simulink model "D53_LKAS"  (R2018b)
settings: Solver=ode3  StartTime=0.0  StopTime=10.0  FixedStep=0.01  RelTol=1e-3  EnableMultiTasking=on
model workspace (MAT data in the model file):
  MCOS : class17 (value not decoded)
  MCOS : class17 (value not decoded)
  MCOS : class17 (value not decoded)
  MCOS : class17 (value not decoded)
  MCOS : class17 (value not decoded)
  MCOS : class17 (value not decoded)
  MCOS : class17 (value not decoded)
  MCOS : class17 (value not decoded)
  MCOS : class17 (value not decoded)
  MCOS : class17 (value not decoded)
  MCOS : class17 (value not decoded)
  MCOS : class17 (value not decoded)
  MCOS : class17 (value not decoded)
  MCOS : class17 (value not decoded)
  MCOS : class17 (value not decoded)
  MCOS : class17 (value not decoded)
  MCOS : class17 (value not decoded)
  MCOS : class17 (value not decoded)
  MCOS : class17 (value not decoded)
  MCOS : class17 (value not decoded)
  MCOS : class17 (value not decoded)
  MCOS : class17 (value not decoded)
  MCOS : class17 (value not decoded)
  MCOS : class17 (value not decoded)
  MCOS : class17 (value not decoded)
  MCOS : class17 (value not decoded)
  MCOS : class17 (value not decoded)
  MCOS : class17 (value not decoded)
  MCOS : class17 (value not decoded)
  MCOS : class17 (value not decoded)
  MCOS : class17 (value not decoded)
  MCOS : class17 (value not decoded)
  MCOS : class17 (value not decoded)
  MCOS : class17 (value not decoded)
  MCOS : class17 (value not decoded)
  MCOS : class17 (value not decoded)
  MCOS : class17 (value not decoded)
  MCOS : class17 (value not decoded)
  MCOS : class17 (value not decoded)
  MCOS : class17 (value not decoded)
  MCOS : class17 (value not decoded)
  MCOS : class17 (value not decoded)
  MCOS : class17 (value not decoded)
  MCOS : class17 (value not decoded)
  MCOS : class17 (value not decoded)
  MCOS : class17 (value not decoded)
  MCOS : class17 (value not decoded)
  MCOS : class17 (value not decoded)
  MCOS : class17 (value not decoded)
  MCOS : class17 (value not decoded)
  MCOS : class17 (value not decoded)
  MCOS : class17 (value not decoded)
  MCOS : class17 (value not decoded)
  MCOS : class17 (value not decoded)
  MCOS : class17 (value not decoded)
  MCOS : class17 (value not decoded)
  MCOS : class17 (value not decoded)
  MCOS : class17 (value not decoded)
  MCOS : class17 (value not decoded)
  MCOS : class17 (value not decoded)
  MCOS : class17 (value not decoded)
  MCOS : class17 (value not decoded)
  MCOS : class17 (value not decoded)
  MCOS : class17 (value not decoded)
  MCOS : class17 (value not decoded)
  MCOS : class17 (value not decoded)
  MCOS : class17 (value not decoded)
  MCOS : class17 (value not decoded)
  MCOS : class17 (value not decoded)
  MCOS : class17 (value not decoded)
  MCOS : class17 (value not decoded)
  MCOS : class17 (value not decoded)
  MCOS : class17 (value not decoded)
  MCOS : class17 (value not decoded)
  MCOS : class17 (value not decoded)
  MCOS : class17 (value not decoded)
  MCOS : class17 (value not decoded)
  MCOS : class17 (value not decoded)
  MCOS : class17 (value not decoded)
  MCOS : class17 (value not decoded)
  MCOS : class17 (value not decoded)
  MCOS : class17 (value not decoded)
  MCOS : class17 (value not decoded)
  MCOS : class17 (value not decoded)
  MCOS : class17 (value not decoded)
  MCOS : class17 (value not decoded)
  MCOS : class17 (value not decoded)
  MCOS : class17 (value not decoded)
  MCOS : class17 (value not decoded)
values from neighbouring files (symbols this model uses):
  C = who    [Data_Made_Data.m]    (also in Data_Make_Data.m; Data_Process.m)
  LKA_SampleTime = Simulink.Parameter    [Model_NoProtect_Script.m]
  Monitor = find_system(strcat(filename,'/CAN Monitor (CANMon)/Monitor'),'SearchDepth',1,'BlockType','From')    [UpdateMon.m]    (also in UpdateMonAuto.m = find_system(strcat(scriptfile,'/CAN Monitor (CANMon)/Monitor; UpdateMonMdb.m; Update_MonAuto.m = find_system(strcat(scriptfile,'/CAN Monitor (CANMon)/Monitor; Update_MonMdb.m)
undefined symbols (not defined in the file or in its folder): LKA_CarWidth, LKA_StrRatio_C, LKA_Veh2CamL_C, LKA_Veh2CamW_C, LKA_WhlBaseL_C, LL_CompSWA_C, LL_CrvtPrvwT_C, LL_DesDvt_C, LL_DvtComp_C, LL_DvtPrvwT_C, LL_DvtSpdDet_vDvtSpdMin_C, LL_HdAgExT_C, LL_HdAgPrvwT_C, LL_LAccMax_C, LL_LAccRMax_C, LL_LDW_EarliestWarnLine_C, LL_LDW_LatestWarnLine_C, LL_LDWS_SUPPRESS_HEADING, LL_LFClb_TFC_DiffCtlBalance, LL_LFClb_TFC_DiffCtrlMaxSWA, LL_LFClb_TFC_DiffCtrlRatio, LL_LFClb_TFC_facmGainLutGain1_C, LL_LFClb_TFC_facmGainLutGain2_C, LL_LFClb_TFC_facmIntegRatio, LL_LFClb_TFC_facmKlat_C, LL_LFClb_TFC_FfCtlRatio_C, LL_LFClb_TFC_phiIntegCtlMaxSWA_C, LL_LFClb_TFC_tiKlatPrvwT_C, LL_LFClb_TFC_vGainLutVehSpdLwr_C, LL_LFClb_TFC_vGainLutVehSpdUpr_C, LL_LKA_EarliestWarnLine_C, LL_LKA_LatestWarnLine_C, LL_LKAExPrcs_ExitC0Dvt, LL_LKAExPrcs_ExitC0Swt, LL_LKAExPrcs_tiExitTime1, LL_LKAExPrcs_tiExitTime2, LL_LKAExPrcs_tiExitTime3, LL_LKAS_OUT_OF_CONTROL_LAT_VEL, LL_LKAS_OUT_OF_CONTROL_TTLC, LL_LKASWASyn_M0, LL_LKASWASyn_M1, LL_LKASWASyn_M2, LL_LKASWASyn_M3K, LL_LKASWASyn_SWAaddMax, LL_LKASWASyn_T2, LL_LKASWASyn_tiTrqSwaRtTime, LL_LKASWASyn_tiTrqSwaTime, LL_LKASWASyn_TrqMax, LL_LKASWASyn_TrqSwaAddSwt, LL_LKASWASyn_TrqSwaRateDiff, LL_LSpdCompT_C, LL_lStpLngth_C, LL_MAX_DELAY_EPSSTAR_TIME, LL_MAX_DRIVER_TORQUE_DISABLE, LL_MAX_DRIVER_TORQUE_ENABLE, LL_MAX_LANE_WIDTH_DISABLE, LL_MAX_LANE_WIDTH_ENABLE, LL_MAX_LAT_ACC_DISABLE, LL_MAX_LAT_ACC_ENABLE, LL_MAX_LDWS_SPEED_DISABLE ... (+29)
libraries: simulink x134, canmsglib x36, dspstat3 x3, simulink_extras x1
(part 7 of 17)

== system D53_LKAS/Clb/Calibration2/Subsystem2/If Action Subsystem3 ==
  In1 : Inport
  Action Port : ActionPort  ActionType=elseif
  Out1 : Outport
  wires:
  In1/1 -> Out1/1

== system D53_LKAS/Clb/Calibration2/Subsystem2/If Action Subsystem4 ==
  In1 : Inport
  Action Port : ActionPort  ActionType=elseif
  Out1 : Outport
  wires:
  In1/1 -> Out1/1

== system D53_LKAS/Clb/Calibration2/Subsystem2/If Action Subsystem5 ==
  In1 : Inport
  Action Port : ActionPort  ActionType=elseif
  Out1 : Outport
  wires:
  In1/1 -> Out1/1

== system D53_LKAS/Clb/Calibration2/Subsystem2/If Action Subsystem6 ==
  In1 : Inport
  Action Port : ActionPort  ActionType=elseif
  Out1 : Outport
  wires:
  In1/1 -> Out1/1

== system D53_LKAS/Clb/Calibration2/Subsystem2/If Action Subsystem7 ==
  In1 : Inport
  Action Port : ActionPort  ActionType=elseif
  Out1 : Outport
  wires:
  In1/1 -> Out1/1

== system D53_LKAS/Clb/Calibration2/Subsystem2/If Action Subsystem8 ==
  In1 : Inport
  Action Port : ActionPort  ActionType=elseif
  Out1 : Outport
  wires:
  In1/1 -> Out1/1

== system D53_LKAS/Clb/Calibration2/Subsystem2/If Action Subsystem9 ==
  In1 : Inport
  Action Port : ActionPort  ActionType=elseif
  Out1 : Outport
  wires:
  In1/1 -> Out1/1

== system D53_LKAS/Clb/Calibration3/Subsystem2/If Action Subsystem ==
  In1 : Inport
  Action Port : ActionPort  ActionType=then
  Out1 : Outport
  wires:
  In1/1 -> Out1/1

== system D53_LKAS/Clb/Calibration3/Subsystem2/If Action Subsystem1 ==
  In1 : Inport
  Action Port : ActionPort  ActionType=elseif
  Out1 : Outport
  wires:
  In1/1 -> Out1/1

== system D53_LKAS/Clb/Calibration3/Subsystem2/If Action Subsystem2 ==
  In1 : Inport
  Action Port : ActionPort  ActionType=elseif
  Out1 : Outport
  wires:
  In1/1 -> Out1/1

== system D53_LKAS/Clb/Calibration3/Subsystem2/If Action Subsystem3 ==
  In1 : Inport
  Action Port : ActionPort  ActionType=elseif
  Out1 : Outport
  wires:
  In1/1 -> Out1/1

== system D53_LKAS/Clb/Calibration3/Subsystem2/If Action Subsystem4 ==
  In1 : Inport
  Action Port : ActionPort  ActionType=elseif
  Out1 : Outport
  wires:
  In1/1 -> Out1/1

== system D53_LKAS/Clb/Calibration3/Subsystem2/If Action Subsystem5 ==
  In1 : Inport
  Action Port : ActionPort  ActionType=elseif
  Out1 : Outport
  wires:
  In1/1 -> Out1/1

== system D53_LKAS/Clb/Calibration3/Subsystem2/If Action Subsystem6 ==
  In1 : Inport
  Action Port : ActionPort  ActionType=elseif
  Out1 : Outport
  wires:
  In1/1 -> Out1/1

== system D53_LKAS/Clb/Calibration3/Subsystem2/If Action Subsystem7 ==
  In1 : Inport
  Action Port : ActionPort  ActionType=elseif
  Out1 : Outport
  wires:
  In1/1 -> Out1/1

== system D53_LKAS/Clb/Calibration3/Subsystem2/If Action Subsystem8 ==
  In1 : Inport
  Action Port : ActionPort  ActionType=elseif
  Out1 : Outport
  wires:
  In1/1 -> Out1/1

== system D53_LKAS/Clb/Calibration3/Subsystem2/If Action Subsystem9 ==
  In1 : Inport
  Action Port : ActionPort  ActionType=elseif
  Out1 : Outport
  wires:
  In1/1 -> Out1/1

== system D53_LKAS/LL/Human Machine Interface (HMI)/Subsystem/Count 10s ==
  Enable : EnablePort  StatesWhenEnabling=reset
  Add : Sum
  Compare To Constant27 : simulink/Logic and Bit Operations/Compare To Constant  relop=>=  const=1000  OutDataTypeStr=boolean
  Constant : Constant  OutDataTypeStr=uint16
  Memory : Memory  InheritSampleTime=on
  Saturation : Saturate  UpperLimit=2100  LowerLimit=0
  Out : Outport  OutputWhenDisabled=reset  InitialOutput=0
  wires:
  Compare To Constant27/1 -> Out/1
  Constant/1 -> Add/1
  Add/1 -> Saturation/1
  Saturation/1 -> Compare To Constant27/1, Memory/1
  Memory/1 -> Add/2

== system D53_LKAS/LL/Human Machine Interface (HMI)/Subsystem/Count 15s ==
  Enable : EnablePort  StatesWhenEnabling=reset
  Add : Sum
  Compare To Constant27 : simulink/Logic and Bit Operations/Compare To Constant  relop=>=  const=1500  OutDataTypeStr=boolean
  Constant : Constant  OutDataTypeStr=uint16
  Memory : Memory  InheritSampleTime=on
  Saturation : Saturate  UpperLimit=2100  LowerLimit=0
  Out : Outport  OutputWhenDisabled=reset  InitialOutput=0
  wires:
  Memory/1 -> Add/2
  Saturation/1 -> Memory/1, Compare To Constant27/1
  Add/1 -> Saturation/1
  Constant/1 -> Add/1
  Compare To Constant27/1 -> Out/1

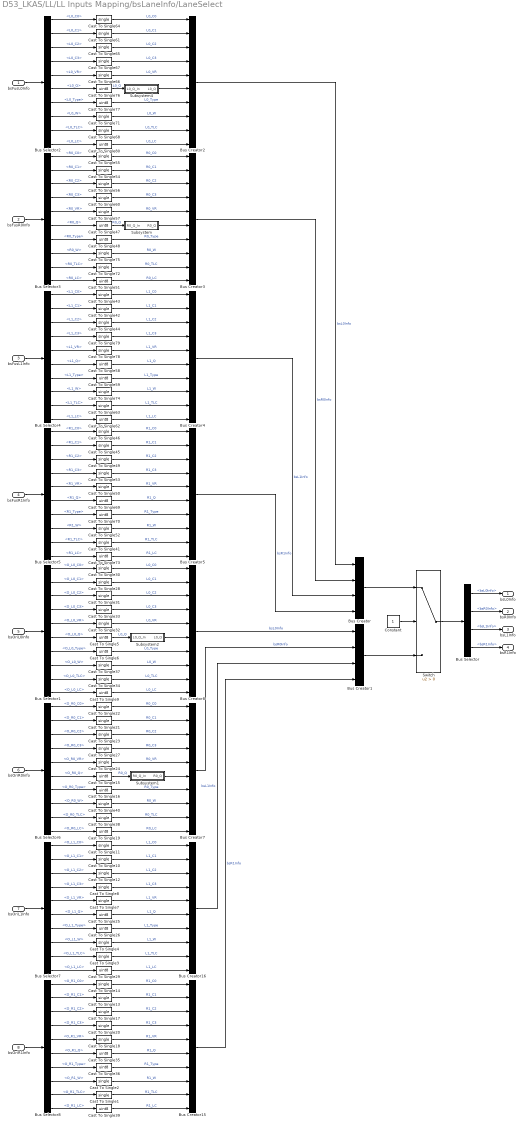
== system D53_LKAS/LL/LL Inputs Mapping/bsLaneInfo/LaneSelect ==
  bsFusL0Info : Inport
  bsFusR0Info : Inport  Port=2
  bsFusL1Info : Inport  Port=3
  bsFusR1Info : Inport  Port=4
  bsOriL0Info : Inport  Port=5
  bsOriR0Info : Inport  Port=6
  bsOriL1Info : Inport  Port=7
  bsOriR1Info : Inport  Port=8
  Bus Creator : BusCreator  Inputs=4
  Bus Creator1 : BusCreator  Inputs=4
  Bus Creator{2..5,7..8,15..16} (8 alike) : BusCreator  Inputs=10
  Bus Selector : BusSelector  OutputSignals=bsL0Info,bsR0Info,bsL1Info,bsR1Info
  Bus Selector1 : BusSelector  OutputSignals=O_L0_C0,O_L0_C1,O_L0_C2,O_L0_C3,O_L0_VR,O_L0_Q,O_L0_Type,O_L0_W,O_L0_TLC,O_L0_LC
  Bus Selector2 : BusSelector  OutputSignals=L0_C0,L0_C1,L0_C2,L0_C3,L0_VR,L0_Q,L0_Type,L0_W,L0_TLC,L0_LC
  Bus Selector3 : BusSelector  OutputSignals=R0_C0,R0_C1,R0_C2,R0_C3,R0_VR,R0_Q,R0_Type,R0_W,R0_TLC,R0_LC
  Bus Selector4 : BusSelector  OutputSignals=L1_C0,L1_C1,L1_C2,L1_C3,L1_VR,L1_Q,L1_Type,L1_W,L1_TLC,L1_LC
  Bus Selector5 : BusSelector  OutputSignals=R1_C0,R1_C1,R1_C2,R1_C3,R1_VR,R1_Q,R1_Type,R1_W,R1_TLC,R1_LC
  Bus Selector6 : BusSelector  OutputSignals=O_R0_C0,O_R0_C1,O_R0_C2,O_R0_C3,O_R0_VR,O_R0_Q,O_R0_Type,O_R0_W,O_R0_TLC,O_R0_LC
  Bus Selector7 : BusSelector  OutputSignals=O_L1_C0,O_L1_C1,O_L1_C2,O_L1_C3,O_L1_VR,O_L1_Q,O_L1_Type,O_L1_W,O_L1_TLC,O_L1_LC
  Bus Selector8 : BusSelector  OutputSignals=O_R1_C0,O_R1_C1,O_R1_C2,O_R1_C3,O_R1_VR,O_R1_Q,O_R1_Type,O_R1_W,O_R1_TLC,O_R1_LC
  Cast To Single{1..4,7..8,10..14,17..18,20..24,27..28,30..34,37..38,40..46,49..50,52..57,60..61,63..68,71..72,74..75,78..79} (56 alike) : DataTypeConversion  OutDataTypeStr=single
  Cast To Single{5..6,9,15..16,19,25..26,29,35..36,39,47..48,51,58..59,62,69..70,73,76..77,80} (24 alike) : DataTypeConversion  OutDataTypeStr=uint8
  Constant : Constant  OutDataTypeStr=uint8
  Subsystem : Subsystem
  Subsystem1 : Subsystem
  Subsystem2 : Subsystem
  Subsystem4 : Subsystem
  Switch : Switch  Criteria=u2 > Threshold
  bsL0Info : Outport
  bsR0Info : Outport  Port=2
  bsL1Info : Outport  Port=3
  bsR1Info : Outport  Port=4
  wires:
  Cast To Single71/1 -> Bus Creator2/8  "L0_W"
  Cast To Single73/1 -> Bus Creator5/10  "R1_LC"
  Cast To Single70/1 -> Bus Creator5/7  "R1_Type"
  Cast To Single69/1 -> Bus Creator5/6  "R1_Q"
  Cast To Single41/1 -> Bus Creator5/9  "R1_TLC"
  Cast To Single53/1 -> Bus Creator5/4  "R1_C3"
  Cast To Single52/1 -> Bus Creator5/8  "R1_W"
  Cast To Single50/1 -> Bus Creator5/5  "R1_VR"
  Cast To Single49/1 -> Bus Creator5/3  "R1_C2"
  Cast To Single46/1 -> Bus Creator5/1  "R1_C0"
  Cast To Single45/1 -> Bus Creator5/2  "R1_C1"
  Cast To Single74/1 -> Bus Creator4/8  "L1_W"
  Cast To Single63/1 -> Bus Creator4/9  "L1_TLC"
  Cast To Single62/1 -> Bus Creator4/10  "L1_LC"
  Cast To Single79/1 -> Bus Creator4/4  "L1_C3"
  Cast To Single78/1 -> Bus Creator4/5  "L1_VR"
  Cast To Single42/1 -> Bus Creator4/2  "L1_C1"
  Cast To Single43/1 -> Bus Creator4/1  "L1_C0"
  Cast To Single59/1 -> Bus Creator4/7  "L1_Type"
  Cast To Single58/1 -> Bus Creator4/6  "L1_Q"
  Cast To Single44/1 -> Bus Creator4/3  "L1_C2"
  Cast To Single75/1 -> Bus Creator3/8  "R0_W"
  Cast To Single72/1 -> Bus Creator3/9  "R0_TLC"
  Cast To Single60/1 -> Bus Creator3/4  "R0_C3"
  Cast To Single57/1 -> Bus Creator3/5  "R0_VR"
  Cast To Single51/1 -> Bus Creator3/10  "R0_LC"
  Cast To Single48/1 -> Bus Creator3/7  "R0_Type"
  Cast To Single47/1 -> Subsystem/1(R0_Q_In)  "R0_Q"
  Cast To Single55/1 -> Bus Creator3/1  "R0_C0"
  Cast To Single54/1 -> Bus Creator3/2  "R0_C1"
  Cast To Single56/1 -> Bus Creator3/3  "R0_C2"
  Cast To Single80/1 -> Bus Creator2/10  "L0_LC"
  Cast To Single77/1 -> Bus Creator2/7  "L0_Type"
  Cast To Single68/1 -> Bus Creator2/9  "L0_TLC"
  Cast To Single76/1 -> Subsystem4/1(L0_Q_In)  "L0_Q"
  Cast To Single64/1 -> Bus Creator2/1  "L0_C0"
  Cast To Single65/1 -> Bus Creator2/3  "L0_C2"
  Cast To Single67/1 -> Bus Creator2/4  "L0_C3"
  Cast To Single66/1 -> Bus Creator2/5  "L0_VR"
  Cast To Single61/1 -> Bus Creator2/2  "L0_C1"
  Bus Creator7/1 -> Bus Creator1/2  "bsR0Info"
  Cast To Single34/1 -> Bus Creator8/9  "L0_TLC"
  Bus Creator15/1 -> Bus Creator1/4  "bsR1Info"
  Cast To Single8/1 -> Bus Creator16/4  "L1_C3"
  Cast To Single29/1 -> Bus Creator16/10  "L1_LC"
  Cast To Single3/1 -> Bus Creator16/9  "L1_TLC"
  Cast To Single18/1 -> Bus Creator15/5  "R1_VR"
  Cast To Single39/1 -> Bus Creator15/10  "R1_LC"
  Cast To Single19/1 -> Bus Creator7/10  "R0_LC"
  Cast To Single12/1 -> Bus Creator16/3  "L1_C2"
  Cast To Single4/1 -> Bus Creator16/8  "L1_W"
  Cast To Single38/1 -> Bus Creator7/9  "R0_TLC"
  Cast To Single11/1 -> Bus Creator16/1  "L1_C0"
  Cast To Single15/1 -> Subsystem1/1(R0_Q_In)  "R0_Q"
  Cast To Single7/1 -> Bus Creator16/5  "L1_VR"
  Cast To Single24/1 -> Bus Creator7/5  "R0_VR"
  Cast To Single20/1 -> Bus Creator15/4  "R1_C3"
  Cast To Single26/1 -> Bus Creator16/7  "L1_Type"
  Cast To Single14/1 -> Bus Creator15/1  "R1_C0"
  Cast To Single13/1 -> Bus Creator15/2  "R1_C1"
  Bus Creator16/1 -> Bus Creator1/3  "bsL1Info"
  Cast To Single23/1 -> Bus Creator7/3  "R0_C2"
  Cast To Single21/1 -> Bus Creator7/2  "R0_C1"
  Cast To Single1/1 -> Bus Creator15/9  "R1_TLC"
  Cast To Single28/1 -> Bus Creator8/2  "L0_C1"
  Cast To Single35/1 -> Bus Creator15/6  "R1_Q"
  Cast To Single16/1 -> Bus Creator7/7  "R0_Type"
  Cast To Single6/1 -> Bus Creator8/7  "L0_Type"
  Cast To Single5/1 -> Subsystem2/1(L0_Q_In)  "L0_Q"
  Cast To Single33/1 -> Bus Creator8/4  "L0_C3"
  Cast To Single30/1 -> Bus Creator8/1  "L0_C0"
  Cast To Single31/1 -> Bus Creator8/3  "L0_C2"
  Cast To Single9/1 -> Bus Creator8/10  "L0_LC"
  Cast To Single36/1 -> Bus Creator15/7  "R1_Type"
  Cast To Single17/1 -> Bus Creator15/3  "R1_C2"
  Cast To Single25/1 -> Bus Creator16/6  "L1_Q"
  Cast To Single22/1 -> Bus Creator7/1  "R0_C0"
  Bus Creator8/1 -> Bus Creator1/1  "bsL0Info"
  Cast To Single40/1 -> Bus Creator7/8  "R0_W"
  Cast To Single37/1 -> Bus Creator8/8  "L0_W"
  Cast To Single32/1 -> Bus Creator8/5  "L0_VR"
  Cast To Single10/1 -> Bus Creator16/2  "L1_C1"
  Cast To Single27/1 -> Bus Creator7/4  "R0_C3"
  Cast To Single2/1 -> Bus Creator15/8  "R1_W"
  bsOriL0Info/1 -> Bus Selector1/1
  Bus Selector1/1 -> Cast To Single30/1  "<O_L0_C0>"
  Bus Selector1/2 -> Cast To Single28/1  "<O_L0_C1>"
  Bus Selector1/3 -> Cast To Single31/1  "<O_L0_C2>"
  Bus Selector1/4 -> Cast To Single33/1  "<O_L0_C3>"
  Bus Selector1/5 -> Cast To Single32/1  "<O_L0_VR>"
  Bus Selector1/6 -> Cast To Single5/1  "<O_L0_Q>"
  Bus Selector1/7 -> Cast To Single6/1  "<O_L0_Type>"
  Bus Selector1/8 -> Cast To Single37/1  "<O_L0_W>"
  Bus Selector1/9 -> Cast To Single34/1  "<O_L0_TLC>"
  Bus Selector1/10 -> Cast To Single9/1  "<O_L0_LC>"
  bsOriR0Info/1 -> Bus Selector6/1
  Bus Selector6/1 -> Cast To Single22/1  "<O_R0_C0>"
  Bus Selector6/2 -> Cast To Single21/1  "<O_R0_C1>"
  Bus Selector6/3 -> Cast To Single23/1  "<O_R0_C2>"
  Bus Selector6/4 -> Cast To Single27/1  "<O_R0_C3>"
  Bus Selector6/5 -> Cast To Single24/1  "<O_R0_VR>"
  Bus Selector6/6 -> Cast To Single15/1  "<O_R0_Q>"
  Bus Selector6/7 -> Cast To Single16/1  "<O_R0_Type>"
  Bus Selector6/8 -> Cast To Single40/1  "<O_R0_W>"
  Bus Selector6/9 -> Cast To Single38/1  "<O_R0_TLC>"
  Bus Selector6/10 -> Cast To Single19/1  "<O_R0_LC>"
  bsOriL1Info/1 -> Bus Selector7/1
  Bus Selector7/1 -> Cast To Single11/1  "<O_L1_C0>"
  Bus Selector7/2 -> Cast To Single10/1  "<O_L1_C1>"
  Bus Selector7/3 -> Cast To Single12/1  "<O_L1_C2>"
  Bus Selector7/4 -> Cast To Single8/1  "<O_L1_C3>"
  Bus Selector7/5 -> Cast To Single7/1  "<O_L1_VR>"
  Bus Selector7/6 -> Cast To Single25/1  "<O_L1_Q>"
  Bus Selector7/7 -> Cast To Single26/1  "<O_L1_Type>"
  Bus Selector7/8 -> Cast To Single4/1  "<O_L1_W>"
  Bus Selector7/9 -> Cast To Single3/1  "<O_L1_TLC>"
  Bus Selector7/10 -> Cast To Single29/1  "<O_L1_LC>"
  bsOriR1Info/1 -> Bus Selector8/1
  Bus Selector8/1 -> Cast To Single14/1  "<O_R1_C0>"
  Bus Selector8/2 -> Cast To Single13/1  "<O_R1_C1>"
  Bus Selector8/3 -> Cast To Single17/1  "<O_R1_C2>"
  Bus Selector8/4 -> Cast To Single20/1  "<O_R1_C3>"
  Bus Selector8/5 -> Cast To Single18/1  "<O_R1_VR>"
  Bus Selector8/6 -> Cast To Single35/1  "<O_R1_Q>"
  Bus Selector8/7 -> Cast To Single36/1  "<O_R1_Type>"
  Bus Selector8/8 -> Cast To Single2/1  "<O_R1_W>"
  Bus Selector8/9 -> Cast To Single1/1  "<O_R1_TLC>"
  Bus Selector8/10 -> Cast To Single39/1  "<O_R1_LC>"
  Bus Creator2/1 -> Bus Creator/1  "bsL0Info"
  Bus Creator3/1 -> Bus Creator/2  "bsR0Info"
  Bus Creator4/1 -> Bus Creator/3  "bsL1Info"
  Bus Creator/1 -> Switch/1
  Bus Creator1/1 -> Switch/3
  Constant/1 -> Switch/2
  Switch/1 -> Bus Selector/1
  Bus Selector4/5 -> Cast To Single78/1  "<L1_VR>"
  Bus Selector4/2 -> Cast To Single42/1  "<L1_C1>"
  Bus Selector3/5 -> Cast To Single57/1  "<R0_VR>"
  Subsystem4/1(L0_Q) -> Bus Creator2/6
  Bus Selector4/1 -> Cast To Single43/1  "<L1_C0>"
  Bus Selector2/4 -> Cast To Single67/1  "<L0_C3>"
  Bus Selector2/6 -> Cast To Single76/1  "<L0_Q>"
  bsFusR1Info/1 -> Bus Selector5/1
  bsFusL1Info/1 -> Bus Selector4/1
  bsFusR0Info/1 -> Bus Selector3/1
  Bus Selector4/7 -> Cast To Single59/1  "<L1_Type>"
  bsFusL0Info/1 -> Bus Selector2/1
  Bus Selector3/10 -> Cast To Single51/1  "<R0_LC>"
  Bus Selector5/10 -> Cast To Single73/1  "<R1_LC>"
  Bus Selector2/3 -> Cast To Single65/1  "<L0_C2>"
  Bus Selector5/1 -> Cast To Single46/1  "<R1_C0>"
  Bus Selector3/8 -> Cast To Single75/1  "<R0_W>"
  Bus Selector3/7 -> Cast To Single48/1  "<R0_Type>"
  Bus Selector3/9 -> Cast To Single72/1  "<R0_TLC>"
  Bus Selector3/3 -> Cast To Single56/1  "<R0_C2>"
  Bus Selector2/10 -> Cast To Single80/1  "<L0_LC>"
  Bus Selector5/7 -> Cast To Single70/1  "<R1_Type>"
  Bus Selector2/9 -> Cast To Single68/1  "<L0_TLC>"
  Bus Selector5/6 -> Cast To Single69/1  "<R1_Q>"
  Bus Selector5/5 -> Cast To Single50/1  "<R1_VR>"
  Bus Selector2/5 -> Cast To Single66/1  "<L0_VR>"
  Bus Selector2/1 -> Cast To Single64/1  "<L0_C0>"
  Bus Selector4/10 -> Cast To Single62/1  "<L1_LC>"
  Bus Selector3/4 -> Cast To Single60/1  "<R0_C3>"
  Bus Selector2/8 -> Cast To Single71/1  "<L0_W>"
  Bus Selector3/2 -> Cast To Single54/1  "<R0_C1>"
  Bus Selector3/1 -> Cast To Single55/1  "<R0_C0>"
  Bus Selector2/2 -> Cast To Single61/1  "<L0_C1>"
  Bus Selector4/4 -> Cast To Single79/1  "<L1_C3>"
  Bus Selector4/6 -> Cast To Single58/1  "<L1_Q>"
  Bus Selector4/9 -> Cast To Single63/1  "<L1_TLC>"
  Bus Selector2/7 -> Cast To Single77/1  "<L0_Type>"
  Subsystem/1(R0_Q) -> Bus Creator3/6
  Bus Selector3/6 -> Cast To Single47/1  "<R0_Q>"
  Bus Selector5/9 -> Cast To Single41/1  "<R1_TLC>"
  Bus Selector5/4 -> Cast To Single53/1  "<R1_C3>"
  Bus Creator5/1 -> Bus Creator/4  "bsR1Info"
  Bus Selector5/8 -> Cast To Single52/1  "<R1_W>"
  Bus Selector5/2 -> Cast To Single45/1  "<R1_C1>"
  Bus Selector5/3 -> Cast To Single49/1  "<R1_C2>"
  Bus Selector4/8 -> Cast To Single74/1  "<L1_W>"
  Bus Selector4/3 -> Cast To Single44/1  "<L1_C2>"
  Bus Selector/1 -> bsL0Info/1  "<bsL0Info>"
  Bus Selector/2 -> bsR0Info/1  "<bsR0Info>"
  Bus Selector/3 -> bsL1Info/1  "<bsL1Info>"
  Bus Selector/4 -> bsR1Info/1  "<bsR1Info>"
  Subsystem2/1(L0_Q) -> Bus Creator8/6
  Subsystem1/1(R0_Q) -> Bus Creator7/6

== system D53_LKAS/LL/LL Inputs Mapping/bsLaneInfo/LanesReconstruct  ==
  bsL0Info : Inport
  bsR0Info : Inport  Port=2
  bsL1Info : Inport  Port=3
  bsR1Info : Inport  Port=4
  Bus Selector5 : BusSelector  OutputSignals=L0_Q
  Bus Selector6 : BusSelector  OutputSignals=R0_Q
  LaneReconstructSM : Stateflow chart  TreatAsAtomicUnit=on
  Left 1Lane Reconstruct (Lft1LaneR) : Subsystem
  Left Lane Reconstruct (LftLaneR) : Subsystem
  Right 1Lane Reconstruct (Rgt1LaneR) : Subsystem
  Right Lane Reconstruct (RgtLaneR) : Subsystem
  RoadSide Offset : Subsystem
  Switch : Switch  Criteria=u2 > Threshold
  Switch1 : Switch  Criteria=u2 > Threshold
  bsL0InfoR : Outport
  bsR0InfoR : Outport  Port=2
  bsL1InfoR : Outport  Port=3
  bsR1InfoR : Outport  Port=4
  wires:
  RoadSide Offset/2(bsR0Infoout) -> Bus Selector6/1, Left Lane Reconstruct (LftLaneR)/2(bsR0Info), Right Lane Reconstruct (RgtLaneR)/2(bsR0Info), Switch/1
  RoadSide Offset/1(bsL0Infoout) -> Bus Selector5/1, Right Lane Reconstruct (RgtLaneR)/1(bsL0Info), Switch1/1, Left Lane Reconstruct (LftLaneR)/3(bsL0Info)
  bsL0Info/1 -> RoadSide Offset/1(bsL0Info)
  bsR0Info/1 -> RoadSide Offset/2(bsR0Info)
  [LftFlg] -> Switch1/2
  [RgtFlg] -> Switch/2
  [LftFlg] -> Left 1Lane Reconstruct (Lft1LaneR)/1(stFlag)
  [RgtFlg] -> Right 1Lane Reconstruct (Rgt1LaneR)/1(stFlag)
  Left 1Lane Reconstruct (Lft1LaneR)/1(bsL1InfoR) -> bsL1InfoR/1
  Right 1Lane Reconstruct (Rgt1LaneR)/1(bsL1InfoR) -> bsR1InfoR/1
  bsR1Info/1 -> Right 1Lane Reconstruct (Rgt1LaneR)/2(bsR1Info)
  LaneReconstructSM/3(LaneRSM_stRgtFlg) -> [RgtFlg]
  LaneReconstructSM/2(LaneRSM_stLftFlg) -> [LftFlg]
  LaneReconstructSM/1(LaneRSM_stRoadFlg) -> [RoadFlg]
  Switch1/1 -> bsL0InfoR/1
  Switch/1 -> bsR0InfoR/1
  Right Lane Reconstruct (RgtLaneR)/1(bsR0InfoR) -> Switch/3
  Left Lane Reconstruct (LftLaneR)/1(bsL0InfoR) -> Switch1/3
  RoadSide Offset/3(lRoadW) -> Right Lane Reconstruct (RgtLaneR)/3(lRoadW), Left Lane Reconstruct (LftLaneR)/1(lRoadW), [RoadWidth]
  Bus Selector5/1 -> LaneReconstructSM/1(LaneRSM_stL0Ql)  "<L0_Q>"
  Bus Selector6/1 -> LaneReconstructSM/2(LaneRSM_stR0Ql)  "<R0_Q>"
  bsL1Info/1 -> Left 1Lane Reconstruct (Lft1LaneR)/2(bsL1Info)

== system D53_LKAS/LL/LLOn/LDW/Heading Angle Detection (HdAgDet) ==
  HdAgDet_stLDWActvFlg : Inport
  HdAgDet_phiHdAgLft : Inport  Port=2
  HdAgDet_phiHdAgRgt : Inport  Port=3
  HdAgDet_phiHdAgThres_C : Inport  Port=4
  Constant : Constant  Value=5  OutDataTypeStr=single
  If : If  IfExpression=u1==1  ElseIfExpressions=u1==2
  If Action Subsystem : Subsystem  TreatAsAtomicUnit=on
  If Action Subsystem1 : Subsystem  TreatAsAtomicUnit=on
  If Action Subsystem2 : Subsystem  TreatAsAtomicUnit=on
  Merge : Merge  Inputs=3  InitialOutput=0
  Relational Operator : RelationalOperator  OutDataTypeStr=boolean  RndMeth=Nearest
  Sum Condition : Subsystem
  HdAgDet_stHdAgDetFlg : Outport
  wires:
  Constant/1 -> Sum Condition/2(Sum)
  Relational Operator/1 -> Sum Condition/Enable, Sum Condition/1(In)
  Sum Condition/1(Out) -> HdAgDet_stHdAgDetFlg/1
  HdAgDet_phiHdAgThres_C/1 -> Relational Operator/2
  Merge/1 -> Relational Operator/1
  HdAgDet_stLDWActvFlg/1 -> If/1
  HdAgDet_phiHdAgRgt/1 -> If Action Subsystem1/1(In1)
  HdAgDet_phiHdAgLft/1 -> If Action Subsystem/1(In1)
  If/3 -> If Action Subsystem2/Action
  If Action Subsystem2/1(Out1) -> Merge/3
  If/2 -> If Action Subsystem1/Action
  If Action Subsystem1/1(Out1) -> Merge/2
  If Action Subsystem/1(Out1) -> Merge/1
  If/1 -> If Action Subsystem/Action

== system D53_LKAS/LL/LLOn/LKA/Driver Torque Addition (DTA) ==
  DTA_bsInInfoSyn : Inport
  DTA_bsLFClb : Inport  Port=2
  Bus Selector : BusSelector  OutputSignals=LL_LKASWAClb.LL_LKASWASyn_TrqSwaAddSwt
  Compare To Constant : simulink/Logic and Bit Operations/Compare To Constant  relop=>  const=0  OutDataTypeStr=boolean
  Subsystem : Subsystem
  Subsystem1 : Subsystem
  DTA_phiDTASWACmd : Outport
  DTA_M : Outport  Port=2
  wires:
  Compare To Constant/1 -> Subsystem/Enable
  Bus Selector/1 -> Compare To Constant/1  "<LL_LKASWASyn_TrqSwaAddSwt>"
  Subsystem1/1(Out1) -> DTA_M/1
  Subsystem/1(Out1) -> DTA_phiDTASWACmd/1
  DTA_bsLFClb/1 -> Bus Selector/1, Subsystem/2(DTA_bsLFClb), Subsystem1/2(DTA_bsLFClb)
  DTA_bsInInfoSyn/1 -> Subsystem1/1(DTA_bsInInfoSyn), Subsystem/1(DTA_bsInInfoSyn)
  [LKA_SampleTime] -> Subsystem/3(LKA_SampleTime)

== system D53_LKAS/LL/LLOn/LKA/LKA Exit Processing (LKAExPrcs) ==
  LKAExPrcs_bsInInfoSyn : Inport
  LKAExPrcs_bsLKAInPInfo : Inport  Port=2
  LKAExPrcs_bsLKAClb : Inport  Port=3
  LKAExPrcs_PlanT1 : Inport  Port=4
  Cast To Single : DataTypeConversion  OutDataTypeStr=single
  Exit Time 1 : Subsystem
  Exit Time 2 : Subsystem
  Exit Time 3 : Subsystem
  Fcn : Fcn  Expr=u(3)*(u(3)==1)*3+u(2)*(u(3)==0)*2+u(1)*(u(2)==0&&u(3)==0)
  Logical Operator3 : Logic  Operator=OR  Inputs=3  AllPortsSameDT=off  OutDataTypeStr=boolean
  Mux : Mux  Inputs=3
  LKAExPrcs_stExFlg : Outport
  LKAExPrcs_stExNum : Outport  Port=2
  wires:
  Cast To Single/1 -> Fcn/1
  Fcn/1 -> LKAExPrcs_stExNum/1  "ExNum"
  Mux/1 -> Cast To Single/1
  LKAExPrcs_PlanT1/1 -> Exit Time 3/4(T1), Exit Time 2/4(T1)
  LKAExPrcs_bsLKAClb/1 -> Exit Time 3/3(bsLKAClb), Exit Time 2/2(bsLKAClb), Exit Time 1/2(bsLKAClb)
  LKAExPrcs_bsLKAInPInfo/1 -> Exit Time 1/1(bsLKAInPInfo), Exit Time 2/3(bsLKAInPInfo), Exit Time 3/2(bsLKAInPInfo)
  Exit Time 3/1(Exit3) -> Logical Operator3/3, Mux/3
  Exit Time 2/1(Exit2) -> Logical Operator3/2, Mux/2
  Exit Time 1/1(Exit1) -> Logical Operator3/1, Mux/1
  Logical Operator3/1 -> LKAExPrcs_stExFlg/1
  LKAExPrcs_bsInInfoSyn/1 -> Exit Time 2/1(bsInInfoSyn), Exit Time 3/1(bsInInfoSyn)

== system D53_LKAS/LL/LLOn/LKA/LKA Motion Planning (LKAMP)  ==
  LKAMP_bsInInfoSyn : Inport
  LKAMP_stLKAActvFlg : Inport  Port=2
  LKAMP_bsLKAInPInfo : Inport  Port=3
  LKAMP_bsLKAClb : Inport  Port=4
  LLClb_bsConstantClb : Inport  Port=5
  Add : Sum  OutDataTypeStr=uint8
  Bus Selector : BusSelector  OutputSignals=MPInP_vVehSpdIni
  Bus Selector1 : BusSelector  OutputSignals=bsVehMovInfo.ESC_VehSpd
  Bus Selector2 : BusSelector  OutputSignals=LKA_CarWidth
  Bus Selector3 : BusSelector  OutputSignals=LL_HdAgExT_C,LL_LSpdCompT_C
  Bus Selector4 : BusSelector  OutputSignals=bsVehMovInfo.ESC_VehSpd
  Bus Selector5 : BusSelector  OutputSignals=LW_LaneWidth
  Constant : Constant  OutDataTypeStr=uint8  SampleTime=-1
  Constant19 : Constant  OutDataTypeStr=uint8  SampleTime=-1
  If : If  NumInputs=2  IfExpression=u1==u2  ShowElse=off
  LKA Motion Planning Calculation (LKAMPCal) : Subsystem  Description=|
      | Block Name: LKA Motion Planning Calculation
      | Ab.: LKAMPCal
      | No.: 1.2.3.2
      | Rev: 0.0.1
      | Update Date: 19-3-26
      settings: RTWSystemCode=Nonreusable function
  Memory1 : Memory  InheritSampleTime=on
  Motion Planning Input Processing (MPInP) : Subsystem  Description=|
      | Block Name: Motion Planning Input Processing
      | Ab.: MPInP
      | No.: 1.2.3.1
      | Rev: 0.0.1
      | Update Date: 19-3-26
  Nominal Time Calculation (NomTCalc) : Subsystem  Description=|
      | Block Name: Nominal Time Calculation
      | Ab.: NomTCalc
      | No.: 1.2.3.3
      | Rev: 0.0.1
      | Update Date: 19-3-26
  Saturation1 : Saturate  UpperLimit=5  LowerLimit=0  OutDataTypeStr=uint8
  Saturation6 : Saturate  UpperLimit=2  LowerLimit=0.2
  Steering Wheel Angle Command Calculation (SWACmdCal) : Subsystem  Description=|
      | Block Name: Steering Wheel Angle Command Calculation
      | Ab.: SWACmdCal
      | No.: 1.2.3.4
      | Rev: 0.0.1
      | Update Date: 19-3-26
  Switching Condition (SwtCon) : Subsystem
  LKAMP_phiSWACmd : Outport
  LKAMP_tiT1 : Outport  Port=2
  LKAMP_tiT2 : Outport  Port=3
  wires:
  Bus Selector5/1 -> Switching Condition (SwtCon)/4(SwtCon_lLaneWidth_C)  "<LW_LaneWidth>"
  Saturation6/1 -> LKAMP_tiT1/1
  LKAMP_bsInInfoSyn/1 -> Bus Selector4/1, Bus Selector1/1, Motion Planning Input Processing (MPInP)/4(MPInP_bsInInfoSyn)
  Bus Selector3/2 -> Switching Condition (SwtCon)/7(SwtCon_tiLSpdCompT_C)  "<LL_LSpdCompT_C>"
  LLClb_bsConstantClb/1 -> Bus Selector2/1, LKA Motion Planning Calculation (LKAMPCal)/3(LLClb_bsConstantClb)
  LKAMP_bsLKAInPInfo/1 -> Motion Planning Input Processing (MPInP)/3(MPInP_bsLKAInPInfo), Switching Condition (SwtCon)/2(SwtCon_bsLKAInPInfo), Bus Selector5/1
  Bus Selector2/1 -> Switching Condition (SwtCon)/5(SwtCon_lCarWidth_C)  "<LKA_CarWidth>"
  LKAMP_bsLKAClb/1 -> LKA Motion Planning Calculation (LKAMPCal)/2(LKAMPCal_bsLKAClb), Bus Selector3/1
  LKAMP_stLKAActvFlg/1 -> Motion Planning Input Processing (MPInP)/1(MPInP_stLKAActvFlg), Switching Condition (SwtCon)/1(SwtCon_stLKAActvFlg)
  Bus Selector4/1 -> Switching Condition (SwtCon)/3(SwtCon_vVehSpd)  "<ESC_VehSpd>"
  Bus Selector3/1 -> Switching Condition (SwtCon)/6(SwtCon_tiHdAgExTime_C)  "<LL_HdAgExT_C>"
  Saturation1/1 -> If/1, Memory1/1
  Add/1 -> Saturation1/1
  Constant19/1 -> If/2
  Constant/1 -> Add/1
  Memory1/1 -> Add/2
  If/1 -> LKA Motion Planning Calculation (LKAMPCal)/Action
  LKA Motion Planning Calculation (LKAMPCal)/1(LKAMPCal_bsLKAMPCalOut) -> Steering Wheel Angle Command Calculation (SWACmdCal)/1(SWACmdCal_bsK1K2DetOut)
  Switching Condition (SwtCon)/1(SwtCon_phiHdAgMax) -> Motion Planning Input Processing (MPInP)/2(MPInP_phiHdAgMax)
  Nominal Time Calculation (NomTCalc)/1(NomTCalc_tiNomT) -> Steering Wheel Angle Command Calculation (SWACmdCal)/3(SWACmdCal_tiNomT)
  Bus Selector1/1 -> Nominal Time Calculation (NomTCalc)/1(NomTCalc_vVehSpd)  "<ESC_VehSpd>"
  Bus Selector/1 -> Nominal Time Calculation (NomTCalc)/2(NomTCalc_vVehSpdIni)  "<MPInP_vVehSpdIni>"
  Steering Wheel Angle Command Calculation (SWACmdCal)/1(SWACmdCal_phiSWACmd) -> LKAMP_phiSWACmd/1
  Steering Wheel Angle Command Calculation (SWACmdCal)/2(SWACmdCal_tiT1) -> Saturation6/1
  Motion Planning Input Processing (MPInP)/1(MPInP_bsMPInPInfo) -> LKA Motion Planning Calculation (LKAMPCal)/1(LKAMPCal_bsLKAInPInfo), Bus Selector/1, Steering Wheel Angle Command Calculation (SWACmdCal)/2(SWACmdCal_bsLKAInPInfo)  "LKAMP_bsMPInPInfo"
  Steering Wheel Angle Command Calculation (SWACmdCal)/3(SWACmdCal_tiT2) -> LKAMP_tiT2/1

== system D53_LKAS/LL/LLOn/LKA/LKA SWA Limit (LKASWALim) ==
  LKASWALim_phiTFCSWACmd : Inport
  LKASWALim_Ff : Inport  Port=2
  LKASWALim_bsLKAInPInfo : Inport  Port=3
  LKASWALim_bsLKAClb : Inport  Port=4
  Add : Sum  Inputs=+-+  OutDataTypeStr=single
  Add1 : Sum
  Add2 : Sum
  Bus Selector1 : BusSelector  OutputSignals=LKAInP_phiSWAPos,UndrLim_phiSWAMax,UndrLim_dphiSWARMax
  Bus Selector3 : BusSelector  OutputSignals=LL_CompSWA_C
  Gain1 : Gain  Gain=-1.4  OutDataTypeStr=single
  Gain2 : Gain  Gain=-1  OutDataTypeStr=single
  Gain3 : Gain  Gain=1.4  OutDataTypeStr=single
  "Rate Limiter Dynamic " : Subsystem
  Saturation Dynamic : simulink/Discontinuities/Saturation Dynamic  OutMin=[]  OutMax=[]  OutDataTypeStr=Inherit: Same as second input  OutDataType=fixdt(1, 16)  OutScaling=2^-10  DoSatur=off
  LKASWALim_phiSWACmd : Outport
  wires:
  Add2/1 -> Saturation Dynamic/3
  Add1/1 -> Saturation Dynamic/1
  LKASWALim_Ff/1 -> Add1/1, Add2/1
  Bus Selector1/1 -> Add/3  "<LKAInP_phiSWAPos>"
  LKASWALim_bsLKAInPInfo/1 -> Bus Selector1/1
  Add/1 -> Saturation Dynamic/2
  Gain1/1 -> "Rate Limiter Dynamic "/3(lo)
  Gain2/1 -> Add2/2
  Bus Selector1/3 -> Gain1/1, Gain3/1  "<UndrLim_dphiSWARMax>"
  Bus Selector1/2 -> Gain2/1, Add1/2  "<UndrLim_phiSWAMax>"
  LKASWALim_bsLKAClb/1 -> Bus Selector3/1
  LKASWALim_phiTFCSWACmd/1 -> Add/1
  Bus Selector3/1 -> Add/2  "<LL_CompSWA_C>"
  "Rate Limiter Dynamic "/1(Y) -> LKASWALim_phiSWACmd/1
  Saturation Dynamic/1 -> "Rate Limiter Dynamic "/2(u)
  Gain3/1 -> "Rate Limiter Dynamic "/1(up)

== system D53_LKAS/LL/LLOn/LKA/LKA_Mon ==
  BusLKA : BusCreator  Inputs=3
  LKAMon : Outport
  wires:
  BusLKA/1 -> LKAMon/1  "LKAMon"
  [T1_Mon] -> BusLKA/3  "T1_Mon"
  [LKA_SampleTime_Mon] -> BusLKA/2  "LKA_SampleTime_Mon"
  [ActFlg_Mon] -> BusLKA/1  "ActFlg_Mon"

== system D53_LKAS/LL/LLOn/LKA/Lane Following (LF) ==
  LF_bsInInfoSyn : Inport
  LF_bsLKAInPInfo : Inport  Port=2
  LF_bsLFClb : Inport  Port=3
  LF_bsConstantClb : Inport  Port=4
  Bus Selector4 : BusSelector  OutputSignals=LL_TFCClb
  Preview Information Calculation (PIC) : Subsystem  Description=|
      | Block Name:Preview Information Calculation
      | Ab.: PIC
      | No.: 02.01
      | Rev: 00.00.01
      | Update Date: 19-3-28
  Trajectory Following Control (TFC) : Subsystem  Description=|
      | Block Name:Trajectory Following Control
      | Ab.: TFC
      | No.: 02.02
      | Rev: 00.00.01
      | Update Date: 19-3-28
  LF_phiFfLFSWACmd : Outport
  LF_phiPropSWACmd : Outport  Port=2
  LF_phiIntegSWACmd : Outport  Port=3
  LF_phiDiffSWACmd : Outport  Port=4
  wires:
  LF_bsLKAInPInfo/1 -> Preview Information Calculation (PIC)/1(PIC_bsLKAInPInfo)
  Trajectory Following Control (TFC)/1(TFC_phiFfSWACmd) -> LF_phiFfLFSWACmd/1
  LF_bsInInfoSyn/1 -> Trajectory Following Control (TFC)/2(TFC_bsInInfoSyn)
  Preview Information Calculation (PIC)/1(PIC_bsPrvwInfo) -> Trajectory Following Control (TFC)/1(TFC_bsPrvwInfo)
  Bus Selector4/1 -> Trajectory Following Control (TFC)/3(TFC_bsTFCClb)  "<LL_TFCClb>"
  LF_bsLFClb/1 -> Bus Selector4/1
  LF_bsConstantClb/1 -> Trajectory Following Control (TFC)/4(TFC_bsConstantClb)
  Trajectory Following Control (TFC)/2(TFC_phiPropSWACmd) -> LF_phiPropSWACmd/1
  Trajectory Following Control (TFC)/3(TFC_phiIntegSWACmd) -> LF_phiIntegSWACmd/1
  Trajectory Following Control (TFC)/4(TFC_phiDiffSWACmd) -> LF_phiDiffSWACmd/1

== system D53_LKAS/LL/LLOn/LKA/Plan To LaneFollowing (PTLF) ==
  InP : Inport
  Plan : Inport  Port=2
  T1 : Inport  Port=3
  DrvTrq : Inport  Port=4
  Ff : Inport  Port=5
  P : Inport  Port=6
  I : Inport  Port=7
  D : Inport  Port=8
  Add1 : Sum  Inputs=+-
  Add2 : Sum  Inputs=+-
  Add3 : Sum
  Add4 : Sum  Inputs=+++++
  Add5 : Sum  Inputs=+-
  Bus Selector1 : BusSelector  OutputSignals=Pr_bsPrInfo.bsPrCrvtInfo.crPrvwCrvt
  Bus Selector2 : BusSelector  OutputSignals=Pr_bsPrInfo.bsPrHdAgInfo.phiHdAgLft,Pr_bsPrInfo.bsPrHdAgInfo.phiHdAgRgt
  Constant1 : Constant  Value=0.1  OutDataTypeStr=single
  Constant2 : Constant  OutDataTypeStr=single
  Divide : Product  Inputs=*/
  Divide{1..2,5..7} (5 alike) : Product  Inputs=**
  Divide3 : Product  Inputs=*/
  Divide4 : Product  Inputs=*/
  InsideJudge : Subsystem
  InsideJudge1 : Subsystem
  LowPass : Subsystem
  Saturation : Saturate  UpperLimit=1  LowerLimit=0
  Saturation1 : Saturate  UpperLimit=1  LowerLimit=0
  Saturation2 : Saturate  UpperLimit=1  LowerLimit=0
  Saturation3 : Saturate  UpperLimit=0.004  LowerLimit=-0.004
  Saturation6 : Saturate  LowerLimit=0.2
  Switch : Switch  Criteria=u2 > Threshold
  TickTime (TTime) : Subsystem
      mask Display:
      | port_label('output', 1, 'TTime');
      | color('blue');
      | text(0.98,0.9,'VCDC Block','horizontalAlignment','right');
      | color('black');
      | text(0.5,0.55,'Tick Time','horizontalAlignment','center');
      | text(0.5,0.4,'(TTime)','horizontalAlignment','center');
  TimeGain : Subsystem
  SWACmd : Outport
  tag scope: LKA_SampleTime_Mon=global, T1_Mon=global
  wires:
  InsideJudge1/2(Plan_1) -> [Plan]
  [Time] -> InsideJudge1/6(Time)
  Plan/1 -> InsideJudge1/5(Plan)
  T1/1 -> InsideJudge1/4(T1)
  Bus Selector2/2 -> InsideJudge1/3(HdAgRgt)  "<phiHdAgRgt>"
  Bus Selector2/1 -> InsideJudge1/2(HdAgLft)  "<phiHdAgLft>"
  [ActFlg] -> InsideJudge1/1(Flg)
  InP/1 -> Bus Selector1/1, Bus Selector2/1
  [Time] -> Add1/1
  Add1/1 -> Divide4/1
  [TFC] -> Divide4/2
  [T1] -> Add1/2
  [TFC] -> TimeGain/3(TFC)
  [T1] -> TimeGain/2(T1)
  [Time] -> TimeGain/1(Time)
  Saturation6/1 -> [TFC]
  InsideJudge1/1(T1_1) -> Saturation6/1, [T1], [T1_Mon]
  [T1] -> Divide3/2
  [Time] -> Add2/1
  [Time] -> Divide3/1
  Switch/1 -> Add4/4  "S_Ff"
  InsideJudge/1(Out1) -> Switch/2
  [ActFlg] -> InsideJudge/1(Flg)
  TickTime (TTime)/1(Out1) -> [Time]
  TimeGain/1(Out1) -> Divide5/1
  Divide5/1 -> Switch/1, Switch/3
  Saturation3/1 -> InsideJudge/2(Crvt)
  Bus Selector1/1 -> Saturation3/1  "<crPrvwCrvt>"
  Saturation1/1 -> Divide2/2
  [TFC] -> Divide/2
  Add4/1 -> LowPass/2(u)
  Add2/1 -> Divide/1
  [T1] -> Add2/2
  Divide3/1 -> Saturation/1
  Divide/1 -> Saturation2/1
  Saturation/1 -> Divide6/2
  Constant2/1 -> Add5/1
  Saturation2/1 -> Add5/2, Divide1/1
  [Plan] -> Divide7/1
  Divide6/1 -> Add4/5  "S_DT"
  Add5/1 -> Divide7/2
  Ff/1 -> Divide5/2
  D/1 -> Divide2/1
  DrvTrq/1 -> Divide6/1
  Divide7/1 -> Add4/1  "S_Plan"
  P/1 -> Add3/1
  I/1 -> Add3/2
  Add3/1 -> Divide1/2
  Divide1/1 -> Add4/2  "S_PI"
  Divide4/1 -> Saturation1/1
  Divide2/1 -> Add4/3  "S_D"
  LowPass/1(y) -> SWACmd/1
  [LKA_SampleTime] -> LowPass/3(dT), [LKA_SampleTime_Mon]
  Constant1/1 -> LowPass/1(T)

== system D53_LKAS/LL/LLOn/LKA Input Processing (LKAInP)/Lane Width Calculation (LW) ==
  LW_bsInInfoSyn : Inport
  Abs : Abs
  Abs1 : Abs
  Add : Sum
  Bus Selector : BusSelector  OutputSignals=bsLaneInfo.bsL0Info.L0_C0,bsLaneInfo.bsR0Info.R0_C0
  Saturation : Saturate  UpperLimit=6  LowerLimit=2
  LW_LaneWidth : Outport
  wires:
  Saturation/1 -> LW_LaneWidth/1  "LaneWidth"
  Add/1 -> Saturation/1
  Abs1/1 -> Add/2
  Abs/1 -> Add/1
  Bus Selector/2 -> Abs1/1  "<R0_C0>"
  Bus Selector/1 -> Abs/1  "<L0_C0>"
  LW_bsInInfoSyn/1 -> Bus Selector/1

== system D53_LKAS/LL/LLOn/LKA Input Processing (LKAInP)/Predicted Deviation Calculation (PrDvt) ==
  PrdcDvt_stLKAActvFlg : Inport
  PrdcDvt_bsInInfoSyn : Inport  Port=2
  PrdcDvt_bsPrdcHdAgInfo : Inport  Port=3
  PrdcDvt_bsLKAClb : Inport  Port=4
  Bus Creator1 : BusCreator  Inputs=8
  Bus Selector : BusSelector  OutputSignals=bsLaneInfo.bsL0Info,bsVehMovInfo.ESC_VehSpd,bsLaneInfo.bsR0Info
  Bus Selector1 : BusSelector  OutputSignals=LL_DvtPrvwT_C,LL_DvtComp_C
  Bus Selector2 : BusSelector  OutputSignals=bsLaneInfo.bsL0Info.L0_C0,bsLaneInfo.bsR0Info.R0_C0
  Bus Selector3 : BusSelector  OutputSignals=EnaCClb.LL_DvtComp_C
  Lane Information Selection (LaneInfoSel) : Subsystem
  Lane Information Selection (LaneInfoSel)1 : Subsystem
  Left Front Conner Deviation Calculation (LFCDvtCalc) : Subsystem
  Predicted Deviation Correction (PrdcDvtCor) : Subsystem
  Predicted Deviation of Left Lane Line (PrdcDvtLft) : Subsystem
  Predicted Deviation of Left Line (PrdcDvtLft) : Subsystem
  Predicted Deviation of Right  Line (PrdcDvtRgt) : Subsystem
  Predicted Deviation of Right Lane Line (PrdcDvtRgt) : Subsystem
  Right Front Conner Deviation Calculation (RFCDvtCalc) : Subsystem
  Z Calculation (ZCalc) : Subsystem
  PrdcDvt_bsPrdcDvtInfo : Outport
  wires:
  Lane Information Selection (LaneInfoSel)1/1(LaneInfoSel_facmActvLane) -> Bus Creator1/6  "lDvt"
  Right Front Conner Deviation Calculation (RFCDvtCalc)/1(DvtCalc_lRgtDvt) -> Bus Creator1/8, Lane Information Selection (LaneInfoSel)1/3(LaneInfoSel_facmRgtLane)  "IRgtDvt"
  Left Front Conner Deviation Calculation (LFCDvtCalc)/1(DvtCalc_lLftDvt) -> Bus Creator1/7, Lane Information Selection (LaneInfoSel)1/2(LaneInfoSel_facmLftLane)  "ILftDvt"
  Bus Selector3/1 -> Left Front Conner Deviation Calculation (LFCDvtCalc)/3(LFCDvtCalc_lDvtComp_C), Right Front Conner Deviation Calculation (RFCDvtCalc)/1(RFCDvtCalc_lDvtComp_C)  "<LL_DvtComp_C>"
  [LLClb_bsLLSMConClb] -> Bus Selector3/1
  Bus Selector2/2 -> Right Front Conner Deviation Calculation (RFCDvtCalc)/2(RFCDvtCalc_lDvt)  "<R0_C0>"
  Bus Selector2/1 -> Left Front Conner Deviation Calculation (LFCDvtCalc)/2(LFCDvtCalc_lDvt)  "<L0_C0>"
  Lane Information Selection (LaneInfoSel)/1(LaneInfoSel_facmActvLane) -> Bus Creator1/1  "lPrdcDvt"
  PrdcDvt_stLKAActvFlg/1 -> Lane Information Selection (LaneInfoSel)1/1(LaneInfoSel_stLKAActvFlg), Lane Information Selection (LaneInfoSel)/1(LaneInfoSel_stLKAActvFlg)
  Bus Creator1/1 -> PrdcDvt_bsPrdcDvtInfo/1
  Predicted Deviation of Right  Line (PrdcDvtRgt)/1(PrdcDvtLft_lDvtRgt) -> Bus Creator1/3, Lane Information Selection (LaneInfoSel)/3(LaneInfoSel_facmRgtLane)  "lPrdcDvtRgt"
  Predicted Deviation of Left Line (PrdcDvtLft)/1(PrdcDvtLft_lDvtLft) -> Lane Information Selection (LaneInfoSel)/2(LaneInfoSel_facmLftLane), Bus Creator1/2  "lPrdcDvtLft"
  Predicted Deviation of Left Lane Line (PrdcDvtLft)/1(PrdcDvtLft_lPrdcDvtLft) -> Predicted Deviation of Left Line (PrdcDvtLft)/3(PrdcDvtLft_lPrdcDvtLft), Bus Creator1/4  "lPrvwDvtLft"
  Bus Selector/3 -> Predicted Deviation of Right Lane Line (PrdcDvtRgt)/2(PrdcDvtRgt_bsR0Info)  "<bsR0Info>"
  Bus Selector/2 -> Z Calculation (ZCalc)/1(ZCalc_vVehSpd)  "<ESC_VehSpd>"
  Predicted Deviation of Right Lane Line (PrdcDvtRgt)/1(PrdcDvtRgt_lPrdcDvtRgt) -> Predicted Deviation of Right  Line (PrdcDvtRgt)/3(PrdcDvtLft_lPrdcDvtLft), Bus Creator1/5  "lPrvwDvtRgt"
  Z Calculation (ZCalc)/1(ZCalc_lPrvwDstZ) -> Predicted Deviation Correction (PrdcDvtCor)/2(PrdcDvtCor_lPrvwDstZ), Predicted Deviation of Left Lane Line (PrdcDvtLft)/2(PrdcDvtLft_lPrvwDstZ), Predicted Deviation of Right Lane Line (PrdcDvtRgt)/1(PrdcDvtRgt_lPrvwDstZ)
  PrdcDvt_bsInInfoSyn/1 -> Bus Selector/1, Bus Selector2/1
  Bus Selector/1 -> Predicted Deviation of Left Lane Line (PrdcDvtLft)/1(PrdcDvtLft_bsL0Info)  "<bsL0Info>"
  PrdcDvt_bsPrdcHdAgInfo/1 -> Predicted Deviation of Left Line (PrdcDvtLft)/1(PrdcDvtLft_bsPrdcHdAgInfo), Predicted Deviation of Right  Line (PrdcDvtRgt)/1(PrdcDvtLft_bsPrdcHdAgInfo), Predicted Deviation Correction (PrdcDvtCor)/1(PrdcDvtCor_bsPrdcHdAgInfo), Left Front Conner Deviation Calculation (LFCDvtCalc)/1(PrdcDvt_bsPrHdAgInfo), Right Front Conner Deviation Calculation (RFCDvtCalc)/3(PrdcDvt_bsPrHdAgInfo)
  Predicted Deviation Correction (PrdcDvtCor)/1(PrdcDvtCor_lPrdcDvtCor) -> Predicted Deviation of Left Line (PrdcDvtLft)/2(PrdcDvtLft_lPrdcDvtCor), Predicted Deviation of Right  Line (PrdcDvtRgt)/2(PrdcDvtLft_lPrdcDvtCor)
  PrdcDvt_bsLKAClb/1 -> Bus Selector1/1
  Bus Selector1/1 -> Z Calculation (ZCalc)/2(ZCalc_tiDvtPrvwT_C)  "<LL_DvtPrvwT_C>"
  Bus Selector1/2 -> Predicted Deviation of Right  Line (PrdcDvtRgt)/4(PrdcDvtLft_lDvtComp_C), Predicted Deviation of Left Line (PrdcDvtLft)/4(PrdcDvtLft_lDvtComp_C)  "<LL_DvtComp_C>"

== system D53_LKAS/LL/LLOn/LKA Input Processing (LKAInP)/Predicted Heading Angle Calculation (PrHdAg) ==
  PrHdAg_bsTTLCInfo : Inport
  PrdcHdAg_stLKAActvFlg : Inport  Port=2
  PrHdAg_bsInInfoSyn : Inport  Port=3
  PrHdAg_bsLKAClb : Inport  Port=4
  Add : Sum  OutDataTypeStr=single
  Add1 : Sum  OutDataTypeStr=single
  Bus Creator : BusCreator  Inputs=10
  Bus Selector : BusSelector  OutputSignals=bsLaneInfo.bsL0Info,bsVehMovInfo.ESC_VehSpd,bsLaneInfo.bsR0Info,bsSWAInfo.SW_Angle
  Bus Selector1 : BusSelector  OutputSignals=LL_HdAgPrvwT_C
  Bus Selector2 : BusSelector  OutputSignals=LFTTTLC,RGTTTLC
  Heading Angle (HdAg) : Subsystem
  Lane Information Selection (LaneInfoSel) : Subsystem
  Lane Information Selection (LaneInfoSel)1 : Subsystem
  Min : MinMax  Inputs=2
  Perdicted Heading Angle Compensation (PrdcHdAgComp) : Subsystem
  Perdicted Heading Angle from Right Lane Line (PrdcHdAgRgt) : Subsystem
  Perdicted Heading Angle from Right Lane Line (PrdcHdAgRgt)1 : Subsystem
  Predicted Heading Angle from Left Lane Line (PrdcHdAgtLft) : Subsystem
  Predicted Heading Angle from Left Lane Line (PrdcHdAgtLft)1 : Subsystem
  Saturation : Saturate  UpperLimit=2  LowerLimit=0.5
  Z Calculation (ZCalc) : Subsystem
  Z Calculation (ZCalc)1 : Subsystem
  PrHdAg_bsPrHdAgInfo : Outport
  wires:
  Perdicted Heading Angle from Right Lane Line (PrdcHdAgRgt)1/1(PrdcHdAgRgt_phiPrdcHdAgRgt) -> Bus Creator/10  "phiPrvwHdAgRgt"
  Predicted Heading Angle from Left Lane Line (PrdcHdAgtLft)1/1(PrdcHdAgtLft_phiPrdcHdAgLft) -> Bus Creator/9  "phiPrvwHdAgLft"
  Z Calculation (ZCalc)1/1(ZCalc_lPrvwDstZ) -> Predicted Heading Angle from Left Lane Line (PrdcHdAgtLft)1/2(PrdcHdAgtLft_lPrvwDstZ), Perdicted Heading Angle from Right Lane Line (PrdcHdAgRgt)1/1(PrdcHdAgRgt_lPrvwDstZ)
  Bus Selector1/1 -> Z Calculation (ZCalc)1/2(ZCalc_tiHdAgPrvwT_C)  "<LL_HdAgPrvwT_C>"
  PrHdAg_bsLKAClb/1 -> Bus Selector1/1
  Heading Angle (HdAg)/3(HdAg_phiHdAgRgt) -> Bus Creator/8  "phiHdAgRgt"
  Heading Angle (HdAg)/2(HdAg_phiHdAgLft) -> Bus Creator/7  "phiHdAgLft"
  Heading Angle (HdAg)/1(HdAg_phiHdAg) -> Bus Creator/6  "phiHdAg"
  Saturation/1 -> Perdicted Heading Angle Compensation (PrdcHdAgComp)/3(PrdcHdAgComp_tiHdAgPrvwT_C), Z Calculation (ZCalc)/2(ZCalc_tiHdAgPrvwT_C)
  Bus Selector2/2 -> Min/2  "<RGTTTLC>"
  Bus Selector2/1 -> Min/1  "<LFTTTLC>"
  PrHdAg_bsTTLCInfo/1 -> Bus Selector2/1
  Lane Information Selection (LaneInfoSel)1/1(LaneInfoSel_facmActvLane) -> Bus Creator/2  "phiPrvwTTLCHdAg"
  Bus Selector/1 -> Predicted Heading Angle from Left Lane Line (PrdcHdAgtLft)/1(PrdcHdAgtLft_bsL0Info), Predicted Heading Angle from Left Lane Line (PrdcHdAgtLft)1/1(PrdcHdAgtLft_bsL0Info)  "<bsL0Info>"
  Z Calculation (ZCalc)/1(ZCalc_lPrvwDstZ) -> Predicted Heading Angle from Left Lane Line (PrdcHdAgtLft)/2(PrdcHdAgtLft_lPrvwDstZ), Perdicted Heading Angle from Right Lane Line (PrdcHdAgRgt)/1(PrdcHdAgRgt_lPrvwDstZ)
  Lane Information Selection (LaneInfoSel)/1(LaneInfoSel_facmActvLane) -> Bus Creator/1  "phiPrdcTTLCHdAg"
  PrdcHdAg_stLKAActvFlg/1 -> Lane Information Selection (LaneInfoSel)/1(LaneInfoSel_stLKAActvFlg), Lane Information Selection (LaneInfoSel)1/1(LaneInfoSel_stLKAActvFlg)
  Add1/1 -> Lane Information Selection (LaneInfoSel)/3(LaneInfoSel_facmRgtLane)  "phiPrdcHdAgRgt"
  Add/1 -> Lane Information Selection (LaneInfoSel)/2(LaneInfoSel_facmLftLane)  "phiPrdcHdAgLft"
  Perdicted Heading Angle Compensation (PrdcHdAgComp)/1(PrdcHdAgComp_phiPrdcHdAgComp) -> Add1/2, Bus Creator/5, Add/2  "phiPrdcHdAgComp"
  Predicted Heading Angle from Left Lane Line (PrdcHdAgtLft)/1(PrdcHdAgtLft_phiPrdcHdAgLft) -> Add/1, Bus Creator/3, Lane Information Selection (LaneInfoSel)1/2(LaneInfoSel_facmLftLane)  "phiPrvwTTLCHdAgLft"
  Perdicted Heading Angle from Right Lane Line (PrdcHdAgRgt)/1(PrdcHdAgRgt_phiPrdcHdAgRgt) -> Add1/1, Lane Information Selection (LaneInfoSel)1/3(LaneInfoSel_facmRgtLane), Bus Creator/4  "phiPrvwTTLCHdAgRgt"
  Bus Creator/1 -> PrHdAg_bsPrHdAgInfo/1
  PrHdAg_bsInInfoSyn/1 -> Bus Selector/1, Heading Angle (HdAg)/1(HdAg_bsLaneInfo)
  Bus Selector/2 -> Z Calculation (ZCalc)/1(ZCalc_vVehSpd), Perdicted Heading Angle Compensation (PrdcHdAgComp)/1(PrdcHdAgComp_vVehSpd), Z Calculation (ZCalc)1/1(ZCalc_vVehSpd)  "<ESC_VehSpd>"
  Bus Selector/3 -> Perdicted Heading Angle from Right Lane Line (PrdcHdAgRgt)/2(PrdcHdAgRgt_bsR0Info), Perdicted Heading Angle from Right Lane Line (PrdcHdAgRgt)1/2(PrdcHdAgRgt_bsR0Info)  "<bsR0Info>"
  Bus Selector/4 -> Perdicted Heading Angle Compensation (PrdcHdAgComp)/2(PrdcHdAgComp_phiSWA)  "<SW_Angle>"
  Min/1 -> Saturation/1

== system D53_LKAS/LL/LLOn/LKA Input Processing (LKAInP)/Previewed Curvature (PrCrvt) ==
  PrvwCrvt_stLKAActvFlg : Inport
  PrvwCrvt_bsInInfoSyn : Inport  Port=2
  PrvwCrvt_tiCrvtPrvwT_C : Inport  Port=3
  Bus Creator : BusCreator  Inputs=3
  Bus Selector : BusSelector  OutputSignals=LL_CrvtPrvwT_C
  Bus Selector2 : BusSelector  OutputSignals=bsLaneInfo.bsL0Info,bsVehMovInfo.ESC_VehSpd,bsLaneInfo.bsR0Info
  Curvature Ahead of Left Lane Line (CrvtAhdLft) : Subsystem
  Curvature Ahead of Left Lane Line (CrvtAhdLft)1 : Subsystem
  Lane Information Selection (LaneInfoSel) : Subsystem
  Z Calculation (ZCalc) : Subsystem
  PrvwCrvt_bsPrvwCrvtInfo : Outport
  wires:
  Bus Creator/1 -> PrvwCrvt_bsPrvwCrvtInfo/1
  Lane Information Selection (LaneInfoSel)/1(LaneInfoSel_facmActvLane) -> Bus Creator/1  "crPrvwCrvt"
  Curvature Ahead of Left Lane Line (CrvtAhdLft)1/1(CrvtAhdRgt_crCrvtAhdRgt) -> Bus Creator/3, Lane Information Selection (LaneInfoSel)/3(LaneInfoSel_facmRgtLane)  "crPrvwCrvtRgt"
  Curvature Ahead of Left Lane Line (CrvtAhdLft)/1(CrvtAhdLft_crCrvtAhdLft) -> Lane Information Selection (LaneInfoSel)/2(LaneInfoSel_facmLftLane), Bus Creator/2  "crPrvwCrvtLft"
  PrvwCrvt_stLKAActvFlg/1 -> Lane Information Selection (LaneInfoSel)/1(LaneInfoSel_stLKAActvFlg)
  Bus Selector/1 -> Z Calculation (ZCalc)/2(ZCalc_tiCrvtPrvwT_C)  "<LL_CrvtPrvwT_C>"
  PrvwCrvt_tiCrvtPrvwT_C/1 -> Bus Selector/1
  Bus Selector2/2 -> Z Calculation (ZCalc)/1(ZCalc_vVehSpd)  "<ESC_VehSpd>"
  Bus Selector2/3 -> Curvature Ahead of Left Lane Line (CrvtAhdLft)1/2(CrvtAhdRgt_bsR0Info)  "<bsR0Info>"
  Bus Selector2/1 -> Curvature Ahead of Left Lane Line (CrvtAhdLft)/1(CrvtAhdLft_bsL0Info)  "<bsL0Info>"
  Z Calculation (ZCalc)/1(ZCalc_lPrvwDstZ) -> Curvature Ahead of Left Lane Line (CrvtAhdLft)/2(CrvtAhdLft_lPrvwDstZ), Curvature Ahead of Left Lane Line (CrvtAhdLft)1/1(CrvtAhdRgt_lPrvwDstZ)
  PrvwCrvt_bsInInfoSyn/1 -> Bus Selector2/1
